simulink model "r2daq"  (R2012b)
settings: Solver=FixedStepDiscrete  SolverMode=SingleTasking  StartTime=0.0  StopTime=10.0  RelTol=1e-3
PreLoadFcn:
  | addpath(genpath('../lib/'));
model workspace (MAT data in the model file):
  pd_coeffbanks = 4
  pd_synthconf = 4
  pd_ctrl_reg = 4
  pd_ddc_2nd_stage = 64
  pd_status_reg = 4
  delay_time_pkt_vs_freq_pkt = 1536
  pd_to_status = 16
  pd_quantize = 16
undefined symbols (not defined in the file or in its folder): sfp
libraries: xbsIndex_r4 x1116, filters x8, r2daq_blocks x7, casper_library_misc x6, xps_library x3, synths x1, simulink x1
(part 2 of 14)

== system r2daq/ctrl_signals ==
  master : Inport
  gain : Inport  Port=2
  fft : Inport  Port=3
  ut0 : Inport  Port=4
  Reinterpret{,1..3} (4 alike) : xbsIndex_r4/Reinterpret  force_arith_type=on  arith_type="Signed  (2's comp)"  force_bin_pt=on  bin_pt=4  block_type=reinterpret
  TimeKeep : r2daq_blocks/TimeKeep
  bit0 : xbsIndex_r4/Slice  nbits=1  boolean_output=on  mode=Lower Bit Location + Width  bit1=0  base1=LSB of Input  bit0=0  base0=LSB of Input  dbl_ovrd=off  block_type=slice
  bits0_12 : xbsIndex_r4/Slice  nbits=13  boolean_output=off  mode=Lower Bit Location + Width  bit1=0  base1=LSB of Input  bit0=0  base0=LSB of Input  dbl_ovrd=off  block_type=slice
  bits0_7 : xbsIndex_r4/Slice  nbits=8  boolean_output=off  mode=Lower Bit Location + Width  bit1=0  base1=LSB of Input  bit0=0  base0=LSB of Input  dbl_ovrd=off  block_type=slice
  bits13_25 : xbsIndex_r4/Slice  nbits=13  boolean_output=off  mode=Lower Bit Location + Width  bit1=0  base1=LSB of Input  bit0=13  base0=LSB of Input  dbl_ovrd=off  block_type=slice
  bits16_23 : xbsIndex_r4/Slice  nbits=8  boolean_output=off  mode=Lower Bit Location + Width  bit1=0  base1=LSB of Input  bit0=8  base0=LSB of Input  dbl_ovrd=off  block_type=slice
  bits24_31 : xbsIndex_r4/Slice  nbits=8  boolean_output=off  mode=Lower Bit Location + Width  bit1=0  base1=LSB of Input  bit0=8  base0=LSB of Input  dbl_ovrd=off  block_type=slice
  bits8_15 : xbsIndex_r4/Slice  nbits=8  boolean_output=off  mode=Lower Bit Location + Width  bit1=0  base1=LSB of Input  bit0=8  base0=LSB of Input  dbl_ovrd=off  block_type=slice
  pipeline : Subsystem  AncestorBlock=casper_library_delays/pipeline  mask(pipeline){latency=pd_ctrl_reg}
      mask help:
      | An explicitly laid-out delay line to avoid mapping to SRL16s
      | for use in pipelining to help achieve timing closure.
      mask init:
      | pipeline_init(gcb,'latency',latency);
      settings: AttributesFormatString=Latency = %<latency>
      mask Display:
      | port_label('input', 1, 'd');
      | port_label('output', 1, 'q');
      | disp(['Z^-', num2str(latency)]);
  pipeline1 : Subsystem  AncestorBlock=casper_library_delays/pipeline  mask(pipeline){latency=pd_ctrl_reg}
      mask help:
      | An explicitly laid-out delay line to avoid mapping to SRL16s
      | for use in pipelining to help achieve timing closure.
      mask init:
      | pipeline_init(gcb,'latency',latency);
      settings: AttributesFormatString=Latency = %<latency>
      mask Display:
      | port_label('input', 1, 'd');
      | port_label('output', 1, 'q');
      | disp(['Z^-', num2str(latency)]);
  pipeline2 : Subsystem  AncestorBlock=casper_library_delays/pipeline  mask(pipeline){latency=pd_ctrl_reg}
      mask help:
      | An explicitly laid-out delay line to avoid mapping to SRL16s
      | for use in pipelining to help achieve timing closure.
      mask init:
      | pipeline_init(gcb,'latency',latency);
      settings: AttributesFormatString=Latency = %<latency>
      mask Display:
      | port_label('input', 1, 'd');
      | port_label('output', 1, 'q');
      | disp(['Z^-', num2str(latency)]);
  pipeline3 : Subsystem  AncestorBlock=casper_library_delays/pipeline  mask(pipeline){latency=pd_ctrl_reg}
      mask help:
      | An explicitly laid-out delay line to avoid mapping to SRL16s
      | for use in pipelining to help achieve timing closure.
      mask init:
      | pipeline_init(gcb,'latency',latency);
      settings: AttributesFormatString=Latency = %<latency>
      mask Display:
      | port_label('input', 1, 'd');
      | port_label('output', 1, 'q');
      | disp(['Z^-', num2str(latency)]);
  rst : Outport
  gain_a : Outport  Port=2
  gain_b : Outport  Port=3
  gain_c : Outport  Port=4
  gain_d : Outport  Port=5
  fft_shift_ab : Outport  Port=6
  fft_shift_cd : Outport  Port=7
  unix_time : Outport  Port=8
  wires:
  bits0_12/1 -> fft_shift_ab/1
  Reinterpret2/1 -> gain_c/1
  fft/1 -> pipeline2/1(d)
  Reinterpret1/1 -> gain_b/1
  [rst_gt] -> TimeKeep/1
  bits0_7/1 -> Reinterpret/1
  bits8_15/1 -> Reinterpret1/1
  bits16_23/1 -> Reinterpret2/1
  bits24_31/1 -> Reinterpret3/1
  master/1 -> pipeline/1(d)
  bits13_25/1 -> fft_shift_cd/1
  gain/1 -> pipeline1/1(d)
  Reinterpret/1 -> gain_a/1
  bit0/1 -> rst/1, [rst_gt]
  pipeline/1(q) -> bit0/1
  TimeKeep/1 -> unix_time/1
  pipeline3/1(q) -> TimeKeep/2
  pipeline1/1(q) -> bits16_23/1, bits24_31/1, bits8_15/1, bits0_7/1
  Reinterpret3/1 -> gain_d/1
  pipeline2/1(q) -> bits13_25/1, bits0_12/1
  ut0/1 -> pipeline3/1(d)

== system r2daq/ddc_1st_a ==
  rst : Inport
  sync_in : Inport  Port=2
  din : Inport  Port=3
  gain : Inport  Port=4
  DigitalDownConverterExt : r2daq_blocks/DigitalDownConverterExt
      link override bus_mul_cosine/a_debus: outputNum=1
      link override bus_mul_cosine/b_debus: outputNum=1
      link override bus_mul_sine/a_debus: outputNum=1
      link override bus_mul_sine/b_debus: outputNum=1
      link override ifir/bus_del1/din_expand: outputNum=1
      link override ifir/bus_del2/din_expand: outputNum=1
      link override ifir/bus_del3/din_expand: outputNum=1
      link override ifir/bus_del4/din_expand: outputNum=1
      link override ifir/bus_del5/din_expand: outputNum=1
      link override ifir/bus_del6/din_expand: outputNum=1
      link override ifir/bus_del7/din_expand: outputNum=1
      link override ifir/bus_mul0/a_debus: outputNum=1
      link override ifir/bus_mul0/b_debus: outputNum=1
      link override ifir/bus_mul1/a_debus: outputNum=1
      link override ifir/bus_mul1/b_debus: outputNum=1
      link override ifir/bus_mul2/a_debus: outputNum=1
      link override ifir/bus_mul2/b_debus: outputNum=1
      link override ifir/bus_mul3/a_debus: outputNum=1
      link override ifir/bus_mul3/b_debus: outputNum=1
      link override ifir/bus_mul4/a_debus: outputNum=1
      link override ifir/bus_mul4/b_debus: outputNum=1
      link override ifir/bus_mul5/a_debus: outputNum=1
      link override ifir/bus_mul5/b_debus: outputNum=1
      link override ifir/bus_mul6/a_debus: outputNum=1
      link override ifir/bus_mul6/b_debus: outputNum=1
      link override ifir/bus_mul7/a_debus: outputNum=1
      link override ifir/bus_mul7/b_debus: outputNum=1
      link override qfir/bus_del1/din_expand: outputNum=1
      link override qfir/bus_del2/din_expand: outputNum=1
      link override qfir/bus_del3/din_expand: outputNum=1
      link override qfir/bus_del4/din_expand: outputNum=1
      link override qfir/bus_del5/din_expand: outputNum=1
      link override qfir/bus_del6/din_expand: outputNum=1
      link override qfir/bus_del7/din_expand: outputNum=1
      link override qfir/bus_mul0/a_debus: outputNum=1
      link override qfir/bus_mul0/b_debus: outputNum=1
      link override qfir/bus_mul1/a_debus: outputNum=1
      link override qfir/bus_mul1/b_debus: outputNum=1
      link override qfir/bus_mul2/a_debus: outputNum=1
      link override qfir/bus_mul2/b_debus: outputNum=1
      link override qfir/bus_mul3/a_debus: outputNum=1
      link override qfir/bus_mul3/b_debus: outputNum=1
      link override qfir/bus_mul4/a_debus: outputNum=1
      link override qfir/bus_mul4/b_debus: outputNum=1
      link override qfir/bus_mul5/a_debus: outputNum=1
      link override qfir/bus_mul5/b_debus: outputNum=1
      link override qfir/bus_mul6/a_debus: outputNum=1
      link override qfir/bus_mul6/b_debus: outputNum=1
      link override qfir/bus_mul7/a_debus: outputNum=1
      link override qfir/bus_mul7/b_debus: outputNum=1
  Gain : r2daq_blocks/Gain
  cb0 : Subsystem  AncestorBlock=filters/coeff_16x8bit_bus  mask(coeff_16x8bit_bus){io_delay=3, sim_in=on, coeff=[0,0,0,0]}
      mask prompts: io_delay "I/O delay for registers"; sim_in "Provide sim input?"; coeff "Coefficients (4 x uint32)"
      mask help:
      | Provides 16x8bit coefficients on a single bus.
      |
      | The coefficients are set in 4x32bit software registers.
      |
      | The I/O delay of the internal registers can be set, as well as an optional simulation input to each.
      mask init:
      | %for ii=0:3
      | %    swr = [gcb sprintf('/g%d',ii)];
      | %    set_param(swr,'sim_port',sim_in);
      | %    set_param(swr,'io_delay',num2str(io_delay));
      | %end
      | coeff_16x8bit_bus_init(gcb,...
      |     'io_delay',io_delay,...
      |     'sim_in',sim_in,...
      |     'coeff',coeff);
      mask Callback sim_in:
      | if strcmpi(get_param(gcb,'sim_in'),'off')
      |     set_param(gcb,'MaskEnables',{'on';'on';'off'});
      | else
      |     set_param(gcb,'MaskEnables',{'on';'on';'on'});
      | end
  cb1 : Subsystem  AncestorBlock=filters/coeff_16x8bit_bus  mask(coeff_16x8bit_bus){io_delay=3, sim_in=on, coeff=[0,0,0,0]}
      mask prompts: io_delay "I/O delay for registers"; sim_in "Provide sim input?"; coeff "Coefficients (4 x uint32)"
      mask help:
      | Provides 16x8bit coefficients on a single bus.
      |
      | The coefficients are set in 4x32bit software registers.
      |
      | The I/O delay of the internal registers can be set, as well as an optional simulation input to each.
      mask init: same as r2daq/ddc_1st_a/cb0
      mask Callback sim_in:
      | if strcmpi(get_param(gcb,'sim_in'),'off')
      |     set_param(gcb,'MaskEnables',{'on';'on';'off'});
      | else
      |     set_param(gcb,'MaskEnables',{'on';'on';'on'});
      | end
  cb2 : Subsystem  AncestorBlock=filters/coeff_16x8bit_bus  mask(coeff_16x8bit_bus){io_delay=3, sim_in=on, coeff=[0,0,0,0]}
      mask prompts: io_delay "I/O delay for registers"; sim_in "Provide sim input?"; coeff "Coefficients (4 x uint32)"
      mask help:
      | Provides 16x8bit coefficients on a single bus.
      |
      | The coefficients are set in 4x32bit software registers.
      |
      | The I/O delay of the internal registers can be set, as well as an optional simulation input to each.
      mask init: same as r2daq/ddc_1st_a/cb0
      mask Callback sim_in:
      | if strcmpi(get_param(gcb,'sim_in'),'off')
      |     set_param(gcb,'MaskEnables',{'on';'on';'off'});
      | else
      |     set_param(gcb,'MaskEnables',{'on';'on';'on'});
      | end
  cb3 : Subsystem  AncestorBlock=filters/coeff_16x8bit_bus  mask(coeff_16x8bit_bus){io_delay=3, sim_in=on, coeff=[0,0,0,0]}
      mask prompts: io_delay "I/O delay for registers"; sim_in "Provide sim input?"; coeff "Coefficients (4 x uint32)"
      mask help:
      | Provides 16x8bit coefficients on a single bus.
      |
      | The coefficients are set in 4x32bit software registers.
      |
      | The I/O delay of the internal registers can be set, as well as an optional simulation input to each.
      mask init: same as r2daq/ddc_1st_a/cb0
      mask Callback sim_in:
      | if strcmpi(get_param(gcb,'sim_in'),'off')
      |     set_param(gcb,'MaskEnables',{'on';'on';'off'});
      | else
      |     set_param(gcb,'MaskEnables',{'on';'on';'on'});
      | end
  cb4 : Subsystem  AncestorBlock=filters/coeff_16x8bit_bus  mask(coeff_16x8bit_bus){io_delay=3, sim_in=on, coeff=[0,0,0,0]}
      mask prompts: io_delay "I/O delay for registers"; sim_in "Provide sim input?"; coeff "Coefficients (4 x uint32)"
      mask help:
      | Provides 16x8bit coefficients on a single bus.
      |
      | The coefficients are set in 4x32bit software registers.
      |
      | The I/O delay of the internal registers can be set, as well as an optional simulation input to each.
      mask init: same as r2daq/ddc_1st_a/cb0
      mask Callback sim_in:
      | if strcmpi(get_param(gcb,'sim_in'),'off')
      |     set_param(gcb,'MaskEnables',{'on';'on';'off'});
      | else
      |     set_param(gcb,'MaskEnables',{'on';'on';'on'});
      | end
  cb5 : Subsystem  AncestorBlock=filters/coeff_16x8bit_bus  mask(coeff_16x8bit_bus){io_delay=3, sim_in=on, coeff=[0,0,0,0]}
      mask prompts: io_delay "I/O delay for registers"; sim_in "Provide sim input?"; coeff "Coefficients (4 x uint32)"
      mask help:
      | Provides 16x8bit coefficients on a single bus.
      |
      | The coefficients are set in 4x32bit software registers.
      |
      | The I/O delay of the internal registers can be set, as well as an optional simulation input to each.
      mask init: same as r2daq/ddc_1st_a/cb0
      mask Callback sim_in:
      | if strcmpi(get_param(gcb,'sim_in'),'off')
      |     set_param(gcb,'MaskEnables',{'on';'on';'off'});
      | else
      |     set_param(gcb,'MaskEnables',{'on';'on';'on'});
      | end
  cb6 : Subsystem  AncestorBlock=filters/coeff_16x8bit_bus  mask(coeff_16x8bit_bus){io_delay=3, sim_in=on, coeff=[0,0,0,0]}
      mask prompts: io_delay "I/O delay for registers"; sim_in "Provide sim input?"; coeff "Coefficients (4 x uint32)"
      mask help:
      | Provides 16x8bit coefficients on a single bus.
      |
      | The coefficients are set in 4x32bit software registers.
      |
      | The I/O delay of the internal registers can be set, as well as an optional simulation input to each.
      mask init: same as r2daq/ddc_1st_a/cb0
      mask Callback sim_in:
      | if strcmpi(get_param(gcb,'sim_in'),'off')
      |     set_param(gcb,'MaskEnables',{'on';'on';'off'});
      | else
      |     set_param(gcb,'MaskEnables',{'on';'on';'on'});
      | end
  cb7 : Subsystem  AncestorBlock=filters/coeff_16x8bit_bus  mask(coeff_16x8bit_bus){io_delay=3, sim_in=on, coeff=[0,0,0,0]}
      mask prompts: io_delay "I/O delay for registers"; sim_in "Provide sim input?"; coeff "Coefficients (4 x uint32)"
      mask help:
      | Provides 16x8bit coefficients on a single bus.
      |
      | The coefficients are set in 4x32bit software registers.
      |
      | The I/O delay of the internal registers can be set, as well as an optional simulation input to each.
      mask init: same as r2daq/ddc_1st_a/cb0
      mask Callback sim_in:
      | if strcmpi(get_param(gcb,'sim_in'),'off')
      |     set_param(gcb,'MaskEnables',{'on';'on';'off'});
      | else
      |     set_param(gcb,'MaskEnables',{'on';'on';'on'});
      | end
  pipeline : Subsystem  AncestorBlock=casper_library_delays/pipeline  mask(pipeline){latency=pd_synthconf}
      mask help:
      | An explicitly laid-out delay line to avoid mapping to SRL16s
      | for use in pipelining to help achieve timing closure.
      mask init:
      | pipeline_init(gcb,'latency',latency);
      settings: AttributesFormatString=Latency = %<latency>
      mask Display:
      | port_label('input', 1, 'd');
      | port_label('output', 1, 'q');
      | disp(['Z^-', num2str(latency)]);
  pipeline1 : Subsystem  AncestorBlock=casper_library_delays/pipeline  mask(pipeline){latency=pd_synthconf}
      mask help:
      | An explicitly laid-out delay line to avoid mapping to SRL16s
      | for use in pipelining to help achieve timing closure.
      mask init:
      | pipeline_init(gcb,'latency',latency);
      settings: AttributesFormatString=Latency = %<latency>
      mask Display:
      | port_label('input', 1, 'd');
      | port_label('output', 1, 'q');
      | disp(['Z^-', num2str(latency)]);
  pipeline10 : Subsystem  AncestorBlock=casper_library_delays/pipeline  mask(pipeline){latency=pd_coeffbanks}
      mask help:
      | An explicitly laid-out delay line to avoid mapping to SRL16s
      | for use in pipelining to help achieve timing closure.
      mask init:
      | pipeline_init(gcb,'latency',latency);
      settings: AttributesFormatString=Latency = %<latency>
      mask Display:
      | port_label('input', 1, 'd');
      | port_label('output', 1, 'q');
      | disp(['Z^-', num2str(latency)]);
  pipeline2 : Subsystem  AncestorBlock=casper_library_delays/pipeline  mask(pipeline){latency=pd_synthconf}
      mask help:
      | An explicitly laid-out delay line to avoid mapping to SRL16s
      | for use in pipelining to help achieve timing closure.
      mask init:
      | pipeline_init(gcb,'latency',latency);
      settings: AttributesFormatString=Latency = %<latency>
      mask Display:
      | port_label('input', 1, 'd');
      | port_label('output', 1, 'q');
      | disp(['Z^-', num2str(latency)]);
  pipeline3 : Subsystem  AncestorBlock=casper_library_delays/pipeline  mask(pipeline){latency=pd_coeffbanks}
      mask help:
      | An explicitly laid-out delay line to avoid mapping to SRL16s
      | for use in pipelining to help achieve timing closure.
      mask init:
      | pipeline_init(gcb,'latency',latency);
      settings: AttributesFormatString=Latency = %<latency>
      mask Display:
      | port_label('input', 1, 'd');
      | port_label('output', 1, 'q');
      | disp(['Z^-', num2str(latency)]);
  pipeline4 : Subsystem  AncestorBlock=casper_library_delays/pipeline  mask(pipeline){latency=pd_coeffbanks}
      mask help:
      | An explicitly laid-out delay line to avoid mapping to SRL16s
      | for use in pipelining to help achieve timing closure.
      mask init:
      | pipeline_init(gcb,'latency',latency);
      settings: AttributesFormatString=Latency = %<latency>
      mask Display:
      | port_label('input', 1, 'd');
      | port_label('output', 1, 'q');
      | disp(['Z^-', num2str(latency)]);
  pipeline5 : Subsystem  AncestorBlock=casper_library_delays/pipeline  mask(pipeline){latency=pd_coeffbanks}
      mask help:
      | An explicitly laid-out delay line to avoid mapping to SRL16s
      | for use in pipelining to help achieve timing closure.
      mask init:
      | pipeline_init(gcb,'latency',latency);
      settings: AttributesFormatString=Latency = %<latency>
      mask Display:
      | port_label('input', 1, 'd');
      | port_label('output', 1, 'q');
      | disp(['Z^-', num2str(latency)]);
  pipeline6 : Subsystem  AncestorBlock=casper_library_delays/pipeline  mask(pipeline){latency=pd_coeffbanks}
      mask help:
      | An explicitly laid-out delay line to avoid mapping to SRL16s
      | for use in pipelining to help achieve timing closure.
      mask init:
      | pipeline_init(gcb,'latency',latency);
      settings: AttributesFormatString=Latency = %<latency>
      mask Display:
      | port_label('input', 1, 'd');
      | port_label('output', 1, 'q');
      | disp(['Z^-', num2str(latency)]);
  pipeline7 : Subsystem  AncestorBlock=casper_library_delays/pipeline  mask(pipeline){latency=pd_coeffbanks}
      mask help:
      | An explicitly laid-out delay line to avoid mapping to SRL16s
      | for use in pipelining to help achieve timing closure.
      mask init:
      | pipeline_init(gcb,'latency',latency);
      settings: AttributesFormatString=Latency = %<latency>
      mask Display:
      | port_label('input', 1, 'd');
      | port_label('output', 1, 'q');
      | disp(['Z^-', num2str(latency)]);
  pipeline8 : Subsystem  AncestorBlock=casper_library_delays/pipeline  mask(pipeline){latency=pd_coeffbanks}
      mask help:
      | An explicitly laid-out delay line to avoid mapping to SRL16s
      | for use in pipelining to help achieve timing closure.
      mask init:
      | pipeline_init(gcb,'latency',latency);
      settings: AttributesFormatString=Latency = %<latency>
      mask Display:
      | port_label('input', 1, 'd');
      | port_label('output', 1, 'q');
      | disp(['Z^-', num2str(latency)]);
  pipeline9 : Subsystem  AncestorBlock=casper_library_delays/pipeline  mask(pipeline){latency=pd_coeffbanks}
      mask help:
      | An explicitly laid-out delay line to avoid mapping to SRL16s
      | for use in pipelining to help achieve timing closure.
      mask init:
      | pipeline_init(gcb,'latency',latency);
      settings: AttributesFormatString=Latency = %<latency>
      mask Display:
      | port_label('input', 1, 'd');
      | port_label('output', 1, 'q');
      | disp(['Z^-', num2str(latency)]);
  synth_input : Subsystem  AncestorBlock=synths/synth_input  mask(synth_input){io_delay=3, sim_in=on, dphi=0, demux_dphi=0, phi0=0}
      mask prompts: io_delay "I/O delay"; sim_in "Sim input?"; dphi "Phase increment per sample"; demux_dphi "Phase increment per demux set"; phi0 "Phase offset"
      mask help:
      | Defines input for synth using a single 32bit software register.
      |
      | I/O delay and optional simulated input for the register are configurable.
      |
      | If simulated input is set, a feed is internally generated using the given parameters for phase increment and offset.
      mask init:
      | synth_input_init(gcb,...
      |     'io_delay',io_delay,...
      |     'sim_in',sim_in,...
      |     'dphi',dphi,...
      |     'demux_dphi',demux_dphi,...
      |     'phi0',phi0);
      mask Callback sim_in:
      | if strcmpi(get_param(gcb,'sim_in'),'on')
      |     set_param(gcb,'MaskEnables',{'on';'on';'on';'on';'on'});
      | else
      |     set_param(gcb,'MaskEnables',{'on';'on';'off';'off';'off'});
      | end
  sync_out : Outport
  dout_c : Outport  Port=2
  wires:
  sync_in/1 -> DigitalDownConverterExt/2
  Gain/2 -> dout_c/1
  DigitalDownConverterExt/2 -> Gain/3
  DigitalDownConverterExt/1 -> Gain/1
  Gain/1 -> sync_out/1
  din/1 -> DigitalDownConverterExt/3
  rst/1 -> DigitalDownConverterExt/1
  synth_input/1(bigdphi) -> pipeline/1(d)
  synth_input/2(smalldphi) -> pipeline1/1(d)
  synth_input/3(phi0) -> pipeline2/1(d)
  cb0/1(coeffbus) -> pipeline3/1(d)
  cb1/1(coeffbus) -> pipeline4/1(d)
  cb2/1(coeffbus) -> pipeline5/1(d)
  cb3/1(coeffbus) -> pipeline6/1(d)
  cb4/1(coeffbus) -> pipeline7/1(d)
  cb5/1(coeffbus) -> pipeline8/1(d)
  cb6/1(coeffbus) -> pipeline9/1(d)
  cb7/1(coeffbus) -> pipeline10/1(d)
  pipeline1/1(q) -> DigitalDownConverterExt/5
  pipeline9/1(q) -> DigitalDownConverterExt/13
  pipeline8/1(q) -> DigitalDownConverterExt/12
  pipeline6/1(q) -> DigitalDownConverterExt/10
  pipeline10/1(q) -> DigitalDownConverterExt/14
  pipeline7/1(q) -> DigitalDownConverterExt/11
  pipeline3/1(q) -> DigitalDownConverterExt/7
  pipeline/1(q) -> DigitalDownConverterExt/4
  pipeline2/1(q) -> DigitalDownConverterExt/6
  pipeline4/1(q) -> DigitalDownConverterExt/8
  pipeline5/1(q) -> DigitalDownConverterExt/9
  gain/1 -> Gain/2

== system r2daq/fft_ctrl ==
  sim_1 : Inport
  io_delay : xbsIndex_r4/Delay  rst=off  infoeditControl=Selection of Reset will increase slice count due to use of real FFs and instead of SRLs  en=off  latency=0  dbl_ovrd=off  reg_retiming=on  block_type=delay
  r2daq_fft_ctrl_user_data_out : xbsIndex_r4/Gateway In  gui_display_data_type=Fixed-point  arith_type=Unsigned  n_bits=32  bin_pt=0  preci_type=Single  exp_width=8  frac_width=24  quantization="Round  (unbiased: +/- Inf)"  overflow=Saturate  period=1  dbl_ovrd=off  timing_constraint=None  locs_specified=off  LOCs={}  UseAsADC=off  ADCChannel='1'  inherit_from_input=off  hdl_port=on  block_type=gatewayin
  reint1 : xbsIndex_r4/Reinterpret  force_arith_type=on  arith_type=Unsigned  force_bin_pt=on  bin_pt=0  block_type=reinterpret
  slice_reg : xbsIndex_r4/Slice  nbits=32  boolean_output=off  mode=Lower Bit Location + Width  bit1=0  base1=MSB of Input  bit0=0  base0=LSB of Input  dbl_ovrd=off  block_type=slice
  in_reg : Outport
  wires:
  r2daq_fft_ctrl_user_data_out/1 -> io_delay/1
  sim_1/1 -> r2daq_fft_ctrl_user_data_out/1
  io_delay/1 -> slice_reg/1
  slice_reg/1 -> reint1/1
  reint1/1 -> in_reg/1

== system r2daq/gain_ctrl ==
  sim_1 : Inport
  io_delay : xbsIndex_r4/Delay  rst=off  infoeditControl=Selection of Reset will increase slice count due to use of real FFs and instead of SRLs  en=off  latency=0  dbl_ovrd=off  reg_retiming=on  block_type=delay
  r2daq_gain_ctrl_user_data_out : xbsIndex_r4/Gateway In  gui_display_data_type=Fixed-point  arith_type=Unsigned  n_bits=32  bin_pt=0  preci_type=Single  exp_width=8  frac_width=24  quantization="Round  (unbiased: +/- Inf)"  overflow=Saturate  period=1  dbl_ovrd=off  timing_constraint=None  locs_specified=off  LOCs={}  UseAsADC=off  ADCChannel='1'  inherit_from_input=off  hdl_port=on  block_type=gatewayin
  reint1 : xbsIndex_r4/Reinterpret  force_arith_type=on  arith_type=Unsigned  force_bin_pt=on  bin_pt=0  block_type=reinterpret
  slice_reg : xbsIndex_r4/Slice  nbits=32  boolean_output=off  mode=Lower Bit Location + Width  bit1=0  base1=MSB of Input  bit0=0  base0=LSB of Input  dbl_ovrd=off  block_type=slice
  in_reg : Outport
  wires:
  r2daq_gain_ctrl_user_data_out/1 -> io_delay/1
  sim_1/1 -> r2daq_gain_ctrl_user_data_out/1
  io_delay/1 -> slice_reg/1
  slice_reg/1 -> reint1/1
  reint1/1 -> in_reg/1

== system r2daq/master_ctrl ==
  sim_1 : Inport
  io_delay : xbsIndex_r4/Delay  rst=off  infoeditControl=Selection of Reset will increase slice count due to use of real FFs and instead of SRLs  en=off  latency=0  dbl_ovrd=off  reg_retiming=on  block_type=delay
  r2daq_master_ctrl_user_data_out : xbsIndex_r4/Gateway In  gui_display_data_type=Fixed-point  arith_type=Unsigned  n_bits=32  bin_pt=0  preci_type=Single  exp_width=8  frac_width=24  quantization="Round  (unbiased: +/- Inf)"  overflow=Saturate  period=1  dbl_ovrd=off  timing_constraint=None  locs_specified=off  LOCs={}  UseAsADC=off  ADCChannel='1'  inherit_from_input=off  hdl_port=on  block_type=gatewayin
  reint1 : xbsIndex_r4/Reinterpret  force_arith_type=on  arith_type=Unsigned  force_bin_pt=on  bin_pt=0  block_type=reinterpret
  slice_reg : xbsIndex_r4/Slice  nbits=32  boolean_output=off  mode=Lower Bit Location + Width  bit1=0  base1=MSB of Input  bit0=0  base0=LSB of Input  dbl_ovrd=off  block_type=slice
  in_reg : Outport
  wires:
  r2daq_master_ctrl_user_data_out/1 -> io_delay/1
  sim_1/1 -> r2daq_master_ctrl_user_data_out/1
  io_delay/1 -> slice_reg/1
  slice_reg/1 -> reint1/1
  reint1/1 -> in_reg/1

== system r2daq/master_status ==
  out_reg : Inport
  assert_reg : xbsIndex_r4/Assert  assert_type=on  type_source=Explicitly  gui_display_data_type=Fixed-point  arith_type=Unsigned  n_bits=32  bin_pt=0  preci_type=Single  exp_width=8  frac_width=24  assert_rate=off  rate_source=Explicitly  period=1  output_port=on  block_type=assert
  cast_gw : xbsIndex_r4/Convert  gui_display_data_type=Fixed-point  arith_type=Unsigned  n_bits=32  bin_pt=0  float_type=Single  exp_bits=8  fraction_bits=24  quantization=Truncate  overflow=Wrap  en=off  latency=0  dbl_ovrd=off  pipeline=off  block_type=convert
  io_delay : xbsIndex_r4/Delay  rst=off  infoeditControl=Selection of Reset will increase slice count due to use of real FFs and instead of SRLs  en=off  latency=0  dbl_ovrd=off  reg_retiming=on  block_type=delay
  r2daq_master_status_user_data_in : xbsIndex_r4/Gateway Out  inherit_from_input=off  hdl_port=on  timing_constraint=None  locs_specified=off  LOCs={}  UseAsDAC=off  DACChannel='1'  block_type=gatewayout
  reint1 : xbsIndex_r4/Reinterpret  force_arith_type=on  arith_type=Unsigned  force_bin_pt=on  bin_pt=0  block_type=reinterpret
  sim_out : Outport
  wires:
  io_delay/1 -> cast_gw/1
  cast_gw/1 -> r2daq_master_status_user_data_in/1
  r2daq_master_status_user_data_in/1 -> sim_out/1
  out_reg/1 -> assert_reg/1
  assert_reg/1 -> reint1/1
  reint1/1 -> io_delay/1

== system r2daq/pipeline ==
  d : Inport
  Register{0..3} (4 alike) : xbsIndex_r4/Register  init=0  rst=off  en=off  dbl_ovrd=off  block_type=register
      Register0 settings: block_version=11.4
      Register1 settings: block_version=11.4
      Register2 settings: block_version=11.4
  q : Outport
  wires:
  Register0/1 -> Register1/1
  Register1/1 -> Register2/1
  Register2/1 -> Register3/1
  d/1 -> Register0/1
  Register3/1 -> q/1

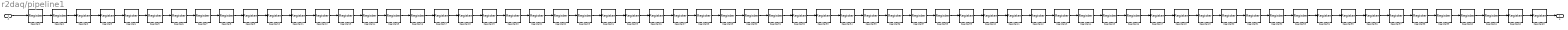
== system r2daq/pipeline1 ==
  d : Inport
  Register{0..63} (64 alike) : xbsIndex_r4/Register  init=0  rst=off  en=off  dbl_ovrd=off  block_type=register
      Register0 settings: block_version=11.4
      Register1 settings: block_version=11.4
      Register2 settings: block_version=11.4
  q : Outport
  wires:
  Register0/1 -> Register1/1
  Register1/1 -> Register2/1
  Register2/1 -> Register3/1
  Register3/1 -> Register4/1
  Register4/1 -> Register5/1
  Register5/1 -> Register6/1
  Register6/1 -> Register7/1
  Register7/1 -> Register8/1
  Register8/1 -> Register9/1
  Register9/1 -> Register10/1
  Register10/1 -> Register11/1
  Register11/1 -> Register12/1
  Register12/1 -> Register13/1
  Register13/1 -> Register14/1
  Register14/1 -> Register15/1
  Register15/1 -> Register16/1
  Register16/1 -> Register17/1
  Register17/1 -> Register18/1
  Register18/1 -> Register19/1
  Register19/1 -> Register20/1
  Register20/1 -> Register21/1
  Register21/1 -> Register22/1
  Register22/1 -> Register23/1
  Register23/1 -> Register24/1
  Register24/1 -> Register25/1
  Register25/1 -> Register26/1
  Register26/1 -> Register27/1
  Register27/1 -> Register28/1
  Register28/1 -> Register29/1
  Register29/1 -> Register30/1
  Register30/1 -> Register31/1
  Register31/1 -> Register32/1
  Register32/1 -> Register33/1
  Register33/1 -> Register34/1
  Register34/1 -> Register35/1
  Register35/1 -> Register36/1
  Register36/1 -> Register37/1
  Register37/1 -> Register38/1
  Register38/1 -> Register39/1
  Register39/1 -> Register40/1
  Register40/1 -> Register41/1
  Register41/1 -> Register42/1
  Register42/1 -> Register43/1
  Register43/1 -> Register44/1
  Register44/1 -> Register45/1
  Register45/1 -> Register46/1
  Register46/1 -> Register47/1
  Register47/1 -> Register48/1
  Register48/1 -> Register49/1
  Register49/1 -> Register50/1
  Register50/1 -> Register51/1
  Register51/1 -> Register52/1
  Register52/1 -> Register53/1
  Register53/1 -> Register54/1
  Register54/1 -> Register55/1
  Register55/1 -> Register56/1
  Register56/1 -> Register57/1
  Register57/1 -> Register58/1
  Register58/1 -> Register59/1
  Register59/1 -> Register60/1
  Register60/1 -> Register61/1
  Register61/1 -> Register62/1
  Register62/1 -> Register63/1
  d/1 -> Register0/1
  Register63/1 -> q/1

== system r2daq/pipeline10 ==
  d : Inport
  Register{0..15} (16 alike) : xbsIndex_r4/Register  init=0  rst=off  en=off  dbl_ovrd=off  block_type=register
      Register0 settings: block_version=11.4
      Register1 settings: block_version=11.4
      Register2 settings: block_version=11.4
  q : Outport
  wires:
  Register0/1 -> Register1/1
  Register1/1 -> Register2/1
  Register2/1 -> Register3/1
  Register3/1 -> Register4/1
  Register4/1 -> Register5/1
  Register5/1 -> Register6/1
  Register6/1 -> Register7/1
  Register7/1 -> Register8/1
  Register8/1 -> Register9/1
  Register9/1 -> Register10/1
  Register10/1 -> Register11/1
  Register11/1 -> Register12/1
  Register12/1 -> Register13/1
  Register13/1 -> Register14/1
  Register14/1 -> Register15/1
  d/1 -> Register0/1
  Register15/1 -> q/1

== system r2daq/pipeline11 ==
  d : Inport
  Register{0..15} (16 alike) : xbsIndex_r4/Register  init=0  rst=off  en=off  dbl_ovrd=off  block_type=register
      Register0 settings: block_version=11.4
      Register1 settings: block_version=11.4
      Register2 settings: block_version=11.4
  q : Outport
  wires:
  Register0/1 -> Register1/1
  Register1/1 -> Register2/1
  Register2/1 -> Register3/1
  Register3/1 -> Register4/1
  Register4/1 -> Register5/1
  Register5/1 -> Register6/1
  Register6/1 -> Register7/1
  Register7/1 -> Register8/1
  Register8/1 -> Register9/1
  Register9/1 -> Register10/1
  Register10/1 -> Register11/1
  Register11/1 -> Register12/1
  Register12/1 -> Register13/1
  Register13/1 -> Register14/1
  Register14/1 -> Register15/1
  d/1 -> Register0/1
  Register15/1 -> q/1

== system r2daq/pipeline12 ==
  d : Inport
  Register{0..15} (16 alike) : xbsIndex_r4/Register  init=0  rst=off  en=off  dbl_ovrd=off  block_type=register
      Register0 settings: block_version=11.4
      Register1 settings: block_version=11.4
      Register2 settings: block_version=11.4
  q : Outport
  wires:
  Register0/1 -> Register1/1
  Register1/1 -> Register2/1
  Register2/1 -> Register3/1
  Register3/1 -> Register4/1
  Register4/1 -> Register5/1
  Register5/1 -> Register6/1
  Register6/1 -> Register7/1
  Register7/1 -> Register8/1
  Register8/1 -> Register9/1
  Register9/1 -> Register10/1
  Register10/1 -> Register11/1
  Register11/1 -> Register12/1
  Register12/1 -> Register13/1
  Register13/1 -> Register14/1
  Register14/1 -> Register15/1
  d/1 -> Register0/1
  Register15/1 -> q/1

== system r2daq/pipeline13 ==
  d : Inport
  Register{0..15} (16 alike) : xbsIndex_r4/Register  init=0  rst=off  en=off  dbl_ovrd=off  block_type=register
      Register0 settings: block_version=11.4
      Register1 settings: block_version=11.4
      Register2 settings: block_version=11.4
  q : Outport
  wires:
  Register0/1 -> Register1/1
  Register1/1 -> Register2/1
  Register2/1 -> Register3/1
  Register3/1 -> Register4/1
  Register4/1 -> Register5/1
  Register5/1 -> Register6/1
  Register6/1 -> Register7/1
  Register7/1 -> Register8/1
  Register8/1 -> Register9/1
  Register9/1 -> Register10/1
  Register10/1 -> Register11/1
  Register11/1 -> Register12/1
  Register12/1 -> Register13/1
  Register13/1 -> Register14/1
  Register14/1 -> Register15/1
  d/1 -> Register0/1
  Register15/1 -> q/1

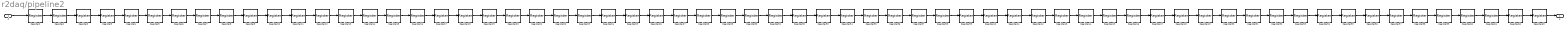
== system r2daq/pipeline2 ==
  d : Inport
  Register{0..63} (64 alike) : xbsIndex_r4/Register  init=0  rst=off  en=off  dbl_ovrd=off  block_type=register
      Register0 settings: block_version=11.4
      Register1 settings: block_version=11.4
      Register2 settings: block_version=11.4
  q : Outport
  wires:
  Register0/1 -> Register1/1
  Register1/1 -> Register2/1
  Register2/1 -> Register3/1
  Register3/1 -> Register4/1
  Register4/1 -> Register5/1
  Register5/1 -> Register6/1
  Register6/1 -> Register7/1
  Register7/1 -> Register8/1
  Register8/1 -> Register9/1
  Register9/1 -> Register10/1
  Register10/1 -> Register11/1
  Register11/1 -> Register12/1
  Register12/1 -> Register13/1
  Register13/1 -> Register14/1
  Register14/1 -> Register15/1
  Register15/1 -> Register16/1
  Register16/1 -> Register17/1
  Register17/1 -> Register18/1
  Register18/1 -> Register19/1
  Register19/1 -> Register20/1
  Register20/1 -> Register21/1
  Register21/1 -> Register22/1
  Register22/1 -> Register23/1
  Register23/1 -> Register24/1
  Register24/1 -> Register25/1
  Register25/1 -> Register26/1
  Register26/1 -> Register27/1
  Register27/1 -> Register28/1
  Register28/1 -> Register29/1
  Register29/1 -> Register30/1
  Register30/1 -> Register31/1
  Register31/1 -> Register32/1
  Register32/1 -> Register33/1
  Register33/1 -> Register34/1
  Register34/1 -> Register35/1
  Register35/1 -> Register36/1
  Register36/1 -> Register37/1
  Register37/1 -> Register38/1
  Register38/1 -> Register39/1
  Register39/1 -> Register40/1
  Register40/1 -> Register41/1
  Register41/1 -> Register42/1
  Register42/1 -> Register43/1
  Register43/1 -> Register44/1
  Register44/1 -> Register45/1
  Register45/1 -> Register46/1
  Register46/1 -> Register47/1
  Register47/1 -> Register48/1
  Register48/1 -> Register49/1
  Register49/1 -> Register50/1
  Register50/1 -> Register51/1
  Register51/1 -> Register52/1
  Register52/1 -> Register53/1
  Register53/1 -> Register54/1
  Register54/1 -> Register55/1
  Register55/1 -> Register56/1
  Register56/1 -> Register57/1
  Register57/1 -> Register58/1
  Register58/1 -> Register59/1
  Register59/1 -> Register60/1
  Register60/1 -> Register61/1
  Register61/1 -> Register62/1
  Register62/1 -> Register63/1
  d/1 -> Register0/1
  Register63/1 -> q/1

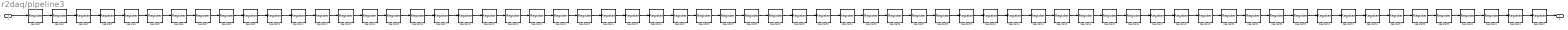
== system r2daq/pipeline3 ==
  d : Inport
  Register{0..63} (64 alike) : xbsIndex_r4/Register  init=0  rst=off  en=off  dbl_ovrd=off  block_type=register
      Register0 settings: block_version=11.4
      Register1 settings: block_version=11.4
      Register2 settings: block_version=11.4
  q : Outport
  wires:
  Register0/1 -> Register1/1
  Register1/1 -> Register2/1
  Register2/1 -> Register3/1
  Register3/1 -> Register4/1
  Register4/1 -> Register5/1
  Register5/1 -> Register6/1
  Register6/1 -> Register7/1
  Register7/1 -> Register8/1
  Register8/1 -> Register9/1
  Register9/1 -> Register10/1
  Register10/1 -> Register11/1
  Register11/1 -> Register12/1
  Register12/1 -> Register13/1
  Register13/1 -> Register14/1
  Register14/1 -> Register15/1
  Register15/1 -> Register16/1
  Register16/1 -> Register17/1
  Register17/1 -> Register18/1
  Register18/1 -> Register19/1
  Register19/1 -> Register20/1
  Register20/1 -> Register21/1
  Register21/1 -> Register22/1
  Register22/1 -> Register23/1
  Register23/1 -> Register24/1
  Register24/1 -> Register25/1
  Register25/1 -> Register26/1
  Register26/1 -> Register27/1
  Register27/1 -> Register28/1
  Register28/1 -> Register29/1
  Register29/1 -> Register30/1
  Register30/1 -> Register31/1
  Register31/1 -> Register32/1
  Register32/1 -> Register33/1
  Register33/1 -> Register34/1
  Register34/1 -> Register35/1
  Register35/1 -> Register36/1
  Register36/1 -> Register37/1
  Register37/1 -> Register38/1
  Register38/1 -> Register39/1
  Register39/1 -> Register40/1
  Register40/1 -> Register41/1
  Register41/1 -> Register42/1
  Register42/1 -> Register43/1
  Register43/1 -> Register44/1
  Register44/1 -> Register45/1
  Register45/1 -> Register46/1
  Register46/1 -> Register47/1
  Register47/1 -> Register48/1
  Register48/1 -> Register49/1
  Register49/1 -> Register50/1
  Register50/1 -> Register51/1
  Register51/1 -> Register52/1
  Register52/1 -> Register53/1
  Register53/1 -> Register54/1
  Register54/1 -> Register55/1
  Register55/1 -> Register56/1
  Register56/1 -> Register57/1
  Register57/1 -> Register58/1
  Register58/1 -> Register59/1
  Register59/1 -> Register60/1
  Register60/1 -> Register61/1
  Register61/1 -> Register62/1
  Register62/1 -> Register63/1
  d/1 -> Register0/1
  Register63/1 -> q/1

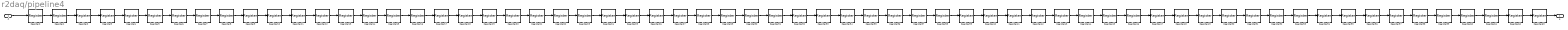
== system r2daq/pipeline4 ==
  d : Inport
  Register{0..63} (64 alike) : xbsIndex_r4/Register  init=0  rst=off  en=off  dbl_ovrd=off  block_type=register
      Register0 settings: block_version=11.4
      Register1 settings: block_version=11.4
      Register2 settings: block_version=11.4
  q : Outport
  wires:
  Register0/1 -> Register1/1
  Register1/1 -> Register2/1
  Register2/1 -> Register3/1
  Register3/1 -> Register4/1
  Register4/1 -> Register5/1
  Register5/1 -> Register6/1
  Register6/1 -> Register7/1
  Register7/1 -> Register8/1
  Register8/1 -> Register9/1
  Register9/1 -> Register10/1
  Register10/1 -> Register11/1
  Register11/1 -> Register12/1
  Register12/1 -> Register13/1
  Register13/1 -> Register14/1
  Register14/1 -> Register15/1
  Register15/1 -> Register16/1
  Register16/1 -> Register17/1
  Register17/1 -> Register18/1
  Register18/1 -> Register19/1
  Register19/1 -> Register20/1
  Register20/1 -> Register21/1
  Register21/1 -> Register22/1
  Register22/1 -> Register23/1
  Register23/1 -> Register24/1
  Register24/1 -> Register25/1
  Register25/1 -> Register26/1
  Register26/1 -> Register27/1
  Register27/1 -> Register28/1
  Register28/1 -> Register29/1
  Register29/1 -> Register30/1
  Register30/1 -> Register31/1
  Register31/1 -> Register32/1
  Register32/1 -> Register33/1
  Register33/1 -> Register34/1
  Register34/1 -> Register35/1
  Register35/1 -> Register36/1
  Register36/1 -> Register37/1
  Register37/1 -> Register38/1
  Register38/1 -> Register39/1
  Register39/1 -> Register40/1
  Register40/1 -> Register41/1
  Register41/1 -> Register42/1
  Register42/1 -> Register43/1
  Register43/1 -> Register44/1
  Register44/1 -> Register45/1
  Register45/1 -> Register46/1
  Register46/1 -> Register47/1
  Register47/1 -> Register48/1
  Register48/1 -> Register49/1
  Register49/1 -> Register50/1
  Register50/1 -> Register51/1
  Register51/1 -> Register52/1
  Register52/1 -> Register53/1
  Register53/1 -> Register54/1
  Register54/1 -> Register55/1
  Register55/1 -> Register56/1
  Register56/1 -> Register57/1
  Register57/1 -> Register58/1
  Register58/1 -> Register59/1
  Register59/1 -> Register60/1
  Register60/1 -> Register61/1
  Register61/1 -> Register62/1
  Register62/1 -> Register63/1
  d/1 -> Register0/1
  Register63/1 -> q/1

== system r2daq/pipeline5 ==
  d : Inport
  Register{0..15} (16 alike) : xbsIndex_r4/Register  init=0  rst=off  en=off  dbl_ovrd=off  block_type=register
      Register0 settings: block_version=11.4
      Register1 settings: block_version=11.4
      Register2 settings: block_version=11.4
  q : Outport
  wires:
  Register0/1 -> Register1/1
  Register1/1 -> Register2/1
  Register2/1 -> Register3/1
  Register3/1 -> Register4/1
  Register4/1 -> Register5/1
  Register5/1 -> Register6/1
  Register6/1 -> Register7/1
  Register7/1 -> Register8/1
  Register8/1 -> Register9/1
  Register9/1 -> Register10/1
  Register10/1 -> Register11/1
  Register11/1 -> Register12/1
  Register12/1 -> Register13/1
  Register13/1 -> Register14/1
  Register14/1 -> Register15/1
  d/1 -> Register0/1
  Register15/1 -> q/1

== system r2daq/pipeline6 ==
  d : Inport
  Register{0..15} (16 alike) : xbsIndex_r4/Register  init=0  rst=off  en=off  dbl_ovrd=off  block_type=register
      Register0 settings: block_version=11.4
      Register1 settings: block_version=11.4
      Register2 settings: block_version=11.4
  q : Outport
  wires:
  Register0/1 -> Register1/1
  Register1/1 -> Register2/1
  Register2/1 -> Register3/1
  Register3/1 -> Register4/1
  Register4/1 -> Register5/1
  Register5/1 -> Register6/1
  Register6/1 -> Register7/1
  Register7/1 -> Register8/1
  Register8/1 -> Register9/1
  Register9/1 -> Register10/1
  Register10/1 -> Register11/1
  Register11/1 -> Register12/1
  Register12/1 -> Register13/1
  Register13/1 -> Register14/1
  Register14/1 -> Register15/1
  d/1 -> Register0/1
  Register15/1 -> q/1

== system r2daq/pipeline7 ==
  d : Inport
  Register{0..15} (16 alike) : xbsIndex_r4/Register  init=0  rst=off  en=off  dbl_ovrd=off  block_type=register
      Register0 settings: block_version=11.4
      Register1 settings: block_version=11.4
      Register2 settings: block_version=11.4
  q : Outport
  wires:
  Register0/1 -> Register1/1
  Register1/1 -> Register2/1
  Register2/1 -> Register3/1
  Register3/1 -> Register4/1
  Register4/1 -> Register5/1
  Register5/1 -> Register6/1
  Register6/1 -> Register7/1
  Register7/1 -> Register8/1
  Register8/1 -> Register9/1
  Register9/1 -> Register10/1
  Register10/1 -> Register11/1
  Register11/1 -> Register12/1
  Register12/1 -> Register13/1
  Register13/1 -> Register14/1
  Register14/1 -> Register15/1
  d/1 -> Register0/1
  Register15/1 -> q/1

== system r2daq/pipeline8 ==
  d : Inport
  Register{0..15} (16 alike) : xbsIndex_r4/Register  init=0  rst=off  en=off  dbl_ovrd=off  block_type=register
      Register0 settings: block_version=11.4
      Register1 settings: block_version=11.4
      Register2 settings: block_version=11.4
  q : Outport
  wires:
  Register0/1 -> Register1/1
  Register1/1 -> Register2/1
  Register2/1 -> Register3/1
  Register3/1 -> Register4/1
  Register4/1 -> Register5/1
  Register5/1 -> Register6/1
  Register6/1 -> Register7/1
  Register7/1 -> Register8/1
  Register8/1 -> Register9/1
  Register9/1 -> Register10/1
  Register10/1 -> Register11/1
  Register11/1 -> Register12/1
  Register12/1 -> Register13/1
  Register13/1 -> Register14/1
  Register14/1 -> Register15/1
  d/1 -> Register0/1
  Register15/1 -> q/1

== system r2daq/pipeline9 ==
  d : Inport
  Register{0..15} (16 alike) : xbsIndex_r4/Register  init=0  rst=off  en=off  dbl_ovrd=off  block_type=register
      Register0 settings: block_version=11.4
      Register1 settings: block_version=11.4
      Register2 settings: block_version=11.4
  q : Outport
  wires:
  Register0/1 -> Register1/1
  Register1/1 -> Register2/1
  Register2/1 -> Register3/1
  Register3/1 -> Register4/1
  Register4/1 -> Register5/1
  Register5/1 -> Register6/1
  Register6/1 -> Register7/1
  Register7/1 -> Register8/1
  Register8/1 -> Register9/1
  Register9/1 -> Register10/1
  Register10/1 -> Register11/1
  Register11/1 -> Register12/1
  Register12/1 -> Register13/1
  Register13/1 -> Register14/1
  Register14/1 -> Register15/1
  d/1 -> Register0/1
  Register15/1 -> q/1
